simulink model "Guidance"  (R2021b)
settings: Solver=VariableStepAuto  StartTime=0.0  StopTime=10.0  RelTol=1e-3
settings Model: DataDictionary=GuidanceDD.sldd  Creator=camil  LastModifiedBy=Paul

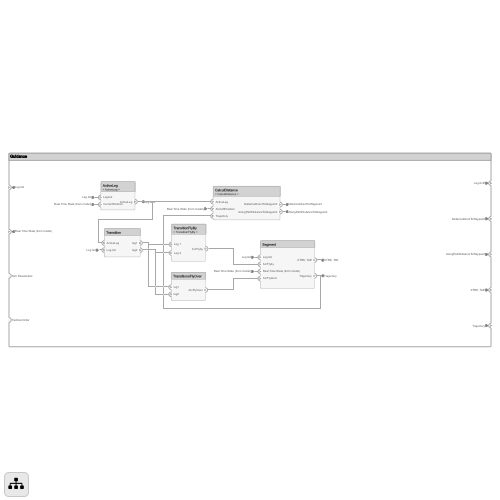
[thumbnail: Simulink's stored preview of the top-level diagram]
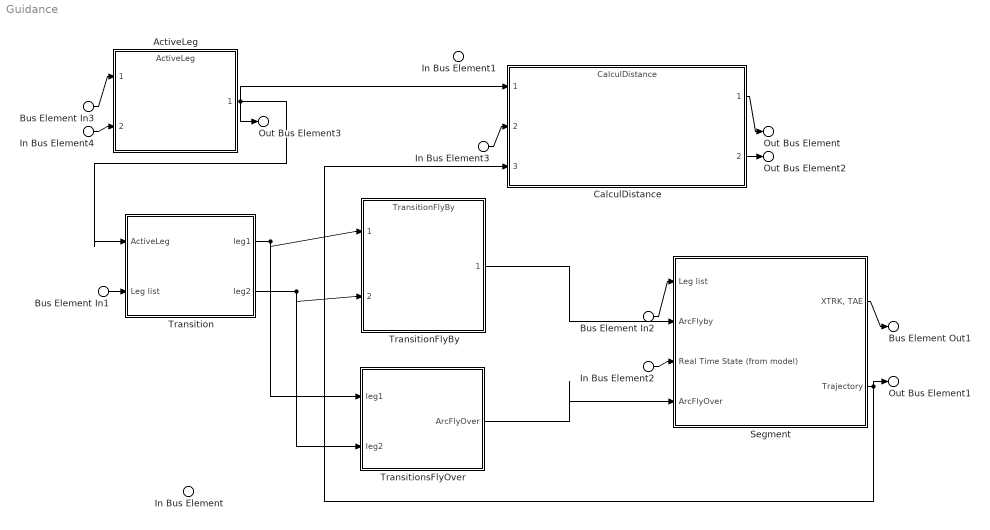
== system Guidance ==
  Bus Element In1 : Inport  RequirementInfo={} %GIDa_7ba553d4_af40_4941_a23b_14e6868a827f  PortName=Leg list
  Bus Element In2 : Inport  PortName=Leg list
  Bus Element In3 : Inport  PortName=Leg list
  In Bus Element3 : Inport  Port=2  PortName=Real Time State (from model)
  In Bus Element2 : Inport  Port=2  PortName=Real Time State (from model)
  In Bus Element4 : Inport  Port=2  PortName=Real Time State (from model)
  In Bus Element : Inport  Port=3  PortName=Sim Parameters
  In Bus Element1 : Inport  Port=4  PortName=Tactical Order
  ActiveLeg : ModelReference  ModelNameDialog=ActiveLeg.slx  SimulationMode=Normal  ModelReferenceVersion=1.2
      settings: PortSchema="{\"entries\":[{\"content\":{\"headerSize\":38,\"margin\":15,\"minimumSpacing\":25,\"sides\":[{\"content\":{\"connectorIds\":[\"In1\",\"In2\"]},\"type\":\"ConnectorPlacement.EquallySpacedRectSide\",\"uuid\":\"40658ef2-5221-47ab-ac15-ac3040122821\"},{\"content\":{\"connectorIds\":[\"Out1\"],\"side\":\"RIGHT\"},\"type\":\"ConnectorPlacement.EquallySpacedRectSide\",\"uuid\":\"9ff354e4-2199-4674-b496-2fe740e12343\"},{\"content\":{\"connectorIds\":[],\"side\":\"TOP\"},\"type\":\"ConnectorPlacement.EquallySpacedRectSide\",\"uuid\":\"dc5fc409-dad0-489a-b972-16c8f80e69f3\"}]},\"type\":\"ConnectorPlacement.EquallySpacedConnector\",\"uuid\":\"f90be94a-f4d5-4fcf-8904-697a887d48e1\"}],\"packageUris\":[\"http://schema.mathworks.com/mf0/Connector/R2020b\"],\"version\":\"1.0\"}"
  CalculDistance : ModelReference  ModelNameDialog=CalculDistance.slx  SimulationMode=Normal  ModelReferenceVersion=1.4
      settings: PortSchema="{\"entries\":[{\"content\":{\"headerSize\":38,\"margin\":15,\"minimumSpacing\":25,\"sides\":[{\"content\":{\"connectorIds\":[\"In1\",\"In2\",\"In3\"]},\"type\":\"ConnectorPlacement.EquallySpacedRectSide\",\"uuid\":\"40658ef2-5221-47ab-ac15-ac3040122821\"},{\"content\":{\"connectorIds\":[\"Out1\",\"Out2\"],\"side\":\"RIGHT\"},\"type\":\"ConnectorPlacement.EquallySpacedRectSide\",\"uuid\":\"9ff354e4-2199-4674-b496-2fe740e12343\"},{\"content\":{\"connectorIds\":[],\"side\":\"TOP\"},\"type\":\"ConnectorPlacement.EquallySpacedRectSide\",\"uuid\":\"dc5fc409-dad0-489a-b972-16c8f80e69f3\"}]},\"type\":\"ConnectorPlacement.EquallySpacedConnector\",\"uuid\":\"f90be94a-f4d5-4fcf-8904-697a887d48e1\"}],\"packageUris\":[\"http://schema.mathworks.com/mf0/Connector/R2020b\"],\"version\":\"1.0\"}"
  Segment : Subsystem
      settings: PortSchema="{\"entries\":[{\"content\":{\"headerSize\":26,\"margin\":15,\"minimumSpacing\":25,\"sides\":[{\"content\":{\"connectorIds\":[\"In1\",\"In2\",\"In3\",\"In4\"]},\"type\":\"ConnectorPlacement.EquallySpacedRectSide\",\"uuid\":\"6b59cfd3-505c-41dc-bf6c-4d82d451ef5d\"},{\"content\":{\"connectorIds\":[\"Out1\",\"Out2\"],\"side\":\"RIGHT\"},\"type\":\"ConnectorPlacement.EquallySpacedRectSide\",\"uuid\":\"f4142fc0-d8fd-40a0-bb01-f33d326facd2\"},{\"content\":{\"connectorIds\":[],\"side\":\"TOP\"},\"type\":\"ConnectorPlacement.EquallySpacedRectSide\",\"uuid\":\"178b855e-eaa2-4b70-a303-d3b7cb6a6ca3\"}]},\"type\":\"ConnectorPlacement.EquallySpacedConnector\",\"uuid\":\"50b576dd-2caa-4080-ba3f-9fa55a69b61e\"}],\"packageUris\":[\"http://schema.mathworks.com/mf0/Connector/R2020b\"],\"version\":\"1.0\"}"
  Transition : Subsystem
      settings: PortSchema="{\"entries\":[{\"content\":{\"headerSize\":26,\"margin\":15,\"minimumSpacing\":25,\"sides\":[{\"content\":{\"connectorIds\":[\"In1\",\"In2\"]},\"type\":\"ConnectorPlacement.EquallySpacedRectSide\",\"uuid\":\"1fe9f491-8940-4068-a798-04a3b940f4fc\"},{\"content\":{\"connectorIds\":[\"Out1\",\"Out2\"],\"side\":\"RIGHT\"},\"type\":\"ConnectorPlacement.EquallySpacedRectSide\",\"uuid\":\"599ca7dc-45bb-4841-abdf-2264bce8800e\"},{\"content\":{\"connectorIds\":[],\"side\":\"TOP\"},\"type\":\"ConnectorPlacement.EquallySpacedRectSide\",\"uuid\":\"c53441a1-491c-45f7-94f0-5f364038b604\"},{\"content\":{\"connectorIds\":[],\"side\":\"BOTTOM\"},\"type\":\"ConnectorPlacement.EquallySpacedRectSide\",\"uuid\":\"eccb86c1-1691-4b5e-892d-381328fb4de3\"}]},\"type\":\"ConnectorPlacement.EquallySpacedConnector\",\"uuid\":\"79cb965a-071d-4caa-a027-7b08a0e7657c\"}],\"packageUris\":[\"http://schema.mathworks.com/mf0/Connector/R2020b\"],\"version\":\"1.0\"}"
  TransitionFlyBy : ModelReference  ModelNameDialog=TransitionFlyBy.slx  SimulationMode=Normal  ModelReferenceVersion=1.5
      settings: PortSchema="{\"entries\":[{\"content\":{\"headerSize\":38,\"margin\":15,\"minimumSpacing\":25,\"sides\":[{\"content\":{\"connectorIds\":[\"In1\",\"In2\"]},\"type\":\"ConnectorPlacement.EquallySpacedRectSide\",\"uuid\":\"527312ce-8ecf-4bed-8b6c-5b5fdf65ac4f\"},{\"content\":{\"connectorIds\":[\"Out1\"],\"side\":\"RIGHT\"},\"type\":\"ConnectorPlacement.EquallySpacedRectSide\",\"uuid\":\"0e60a1e2-e39b-415d-9de3-d9c44bc8d6f1\"},{\"content\":{\"connectorIds\":[],\"side\":\"TOP\"},\"type\":\"ConnectorPlacement.EquallySpacedRectSide\",\"uuid\":\"eb1a168f-e7eb-4116-955a-7fd7ac806224\"}]},\"type\":\"ConnectorPlacement.EquallySpacedConnector\",\"uuid\":\"cb4b2f41-930a-4cb2-9ca3-9a6ca94f5e19\"}],\"packageUris\":[\"http://schema.mathworks.com/mf0/Connector/R2020b\"],\"version\":\"1.0\"}"
  TransitionsFlyOver : Subsystem
      settings: PortSchema="{\"entries\":[{\"content\":{\"headerSize\":26,\"margin\":15,\"minimumSpacing\":25,\"sides\":[{\"content\":{\"connectorIds\":[\"In1\",\"In2\"]},\"type\":\"ConnectorPlacement.EquallySpacedRectSide\",\"uuid\":\"1fe9f491-8940-4068-a798-04a3b940f4fc\"},{\"content\":{\"connectorIds\":[\"Out1\"],\"side\":\"RIGHT\"},\"type\":\"ConnectorPlacement.EquallySpacedRectSide\",\"uuid\":\"599ca7dc-45bb-4841-abdf-2264bce8800e\"},{\"content\":{\"connectorIds\":[],\"side\":\"TOP\"},\"type\":\"ConnectorPlacement.EquallySpacedRectSide\",\"uuid\":\"c53441a1-491c-45f7-94f0-5f364038b604\"}]},\"type\":\"ConnectorPlacement.EquallySpacedConnector\",\"uuid\":\"79cb965a-071d-4caa-a027-7b08a0e7657c\"}],\"packageUris\":[\"http://schema.mathworks.com/mf0/Connector/R2020b\"],\"version\":\"1.0\"}"
  Out Bus Element3 : Outport  PortName=Leg Actif
  Out Bus Element : Outport  Port=2  PortName=DistanceDirectToWaypoint
  Out Bus Element2 : Outport  Port=3  PortName=AlongPathDistanceToWaypoint
  Bus Element Out1 : Outport  RequirementInfo={} %GIDa_9dd73be6_6c5d_401c_be67_fba4302eb24d  Port=4  PortName=XTRK, TAE
  Out Bus Element1 : Outport  Port=5  PortName=Trajectory
  wires:
  Bus Element In1/1 -> Transition/2(Leg list)
  Transition/1(leg1) -> TransitionsFlyOver/1(leg1), TransitionFlyBy/1
  Transition/2(leg2) -> TransitionsFlyOver/2(leg2), TransitionFlyBy/2
  TransitionsFlyOver/1(ArcFlyOver) -> Segment/4(ArcFlyOver)
  Segment/2(Trajectory) -> Out Bus Element1/1, CalculDistance/3
  TransitionFlyBy/1 -> Segment/2(ArcFlyby)
  Bus Element In2/1 -> Segment/1(Leg list)
  In Bus Element2/1 -> Segment/3(Real Time State (from model))
  Segment/1("XTRK, TAE") -> Bus Element Out1/1
  In Bus Element3/1 -> CalculDistance/2
  CalculDistance/2 -> Out Bus Element2/1
  CalculDistance/1 -> Out Bus Element/1
  In Bus Element4/1 -> ActiveLeg/2
  Bus Element In3/1 -> ActiveLeg/1
  ActiveLeg/1 -> Transition/1(ActiveLeg), CalculDistance/1, Out Bus Element3/1

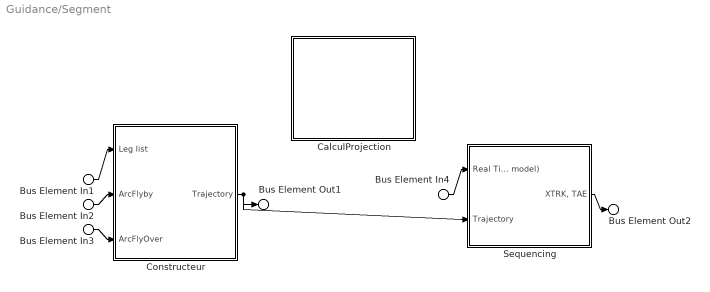
== system Guidance/Segment ==
  Bus Element In1 : Inport  PortName=Leg list
  Bus Element In2 : Inport  Port=2  PortName=ArcFlyby
  Bus Element In4 : Inport  Port=3  PortName=Real Time State (from model)
  Bus Element In3 : Inport  Port=4  PortName=ArcFlyOver
  CalculProjection : Subsystem
      settings: PortSchema="{\"entries\":[{\"content\":{\"headerSize\":26,\"margin\":15,\"minimumSpacing\":25,\"sides\":[{\"content\":{\"connectorIds\":[]},\"type\":\"ConnectorPlacement.EquallySpacedRectSide\",\"uuid\":\"6b59cfd3-505c-41dc-bf6c-4d82d451ef5d\"},{\"content\":{\"connectorIds\":[],\"side\":\"RIGHT\"},\"type\":\"ConnectorPlacement.EquallySpacedRectSide\",\"uuid\":\"f4142fc0-d8fd-40a0-bb01-f33d326facd2\"},{\"content\":{\"connectorIds\":[],\"side\":\"TOP\"},\"type\":\"ConnectorPlacement.EquallySpacedRectSide\",\"uuid\":\"178b855e-eaa2-4b70-a303-d3b7cb6a6ca3\"}]},\"type\":\"ConnectorPlacement.EquallySpacedConnector\",\"uuid\":\"50b576dd-2caa-4080-ba3f-9fa55a69b61e\"}],\"packageUris\":[\"http://schema.mathworks.com/mf0/Connector/R2020b\"],\"version\":\"1.0\"}"
  Constructeur : Subsystem
      settings: PortSchema="{\"entries\":[{\"content\":{\"headerSize\":26,\"margin\":15,\"minimumSpacing\":25,\"sides\":[{\"content\":{\"connectorIds\":[\"In1\",\"In2\",\"In3\"]},\"type\":\"ConnectorPlacement.EquallySpacedRectSide\",\"uuid\":\"1fe9f491-8940-4068-a798-04a3b940f4fc\"},{\"content\":{\"connectorIds\":[\"Out1\"],\"side\":\"RIGHT\"},\"type\":\"ConnectorPlacement.EquallySpacedRectSide\",\"uuid\":\"599ca7dc-45bb-4841-abdf-2264bce8800e\"},{\"content\":{\"connectorIds\":[],\"side\":\"TOP\"},\"type\":\"ConnectorPlacement.EquallySpacedRectSide\",\"uuid\":\"c53441a1-491c-45f7-94f0-5f364038b604\"}]},\"type\":\"ConnectorPlacement.EquallySpacedConnector\",\"uuid\":\"79cb965a-071d-4caa-a027-7b08a0e7657c\"}],\"packageUris\":[\"http://schema.mathworks.com/mf0/Connector/R2020b\"],\"version\":\"1.0\"}"
  Sequencing : Subsystem
      settings: PortSchema="{\"entries\":[{\"content\":{\"headerSize\":26,\"margin\":15,\"minimumSpacing\":25,\"sides\":[{\"content\":{\"connectorIds\":[\"In1\",\"In2\"]},\"type\":\"ConnectorPlacement.EquallySpacedRectSide\",\"uuid\":\"1fe9f491-8940-4068-a798-04a3b940f4fc\"},{\"content\":{\"connectorIds\":[\"Out1\"],\"side\":\"RIGHT\"},\"type\":\"ConnectorPlacement.EquallySpacedRectSide\",\"uuid\":\"599ca7dc-45bb-4841-abdf-2264bce8800e\"},{\"content\":{\"connectorIds\":[],\"side\":\"TOP\"},\"type\":\"ConnectorPlacement.EquallySpacedRectSide\",\"uuid\":\"c53441a1-491c-45f7-94f0-5f364038b604\"}]},\"type\":\"ConnectorPlacement.EquallySpacedConnector\",\"uuid\":\"79cb965a-071d-4caa-a027-7b08a0e7657c\"}],\"packageUris\":[\"http://schema.mathworks.com/mf0/Connector/R2020b\"],\"version\":\"1.0\"}"
  Bus Element Out2 : Outport  PortName=XTRK, TAE
  Bus Element Out1 : Outport  Port=2  PortName=Trajectory
  wires:
  Bus Element In1/1 -> Constructeur/1(Leg list)
  Bus Element In2/1 -> Constructeur/2(ArcFlyby)
  Bus Element In3/1 -> Constructeur/3(ArcFlyOver)
  Constructeur/1(Trajectory) -> Sequencing/2(Trajectory), Bus Element Out1/1
  Bus Element In4/1 -> Sequencing/1(Real Time State (from model))
  Sequencing/1("XTRK, TAE") -> Bus Element Out2/1

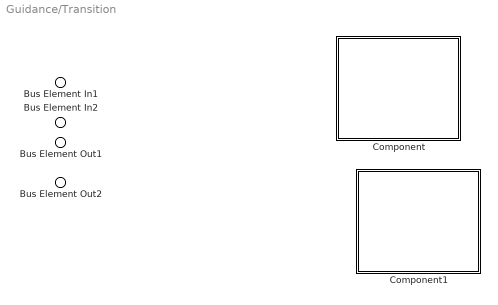
== system Guidance/Transition ==
  Bus Element In1 : Inport  PortName=ActiveLeg
  Bus Element In2 : Inport  Port=2  PortName=Leg list
  Component : Subsystem
      settings: PortSchema="{\"entries\":[{\"content\":{\"headerSize\":26,\"margin\":15,\"minimumSpacing\":25,\"sides\":[{\"content\":{\"connectorIds\":[]},\"type\":\"ConnectorPlacement.EquallySpacedRectSide\",\"uuid\":\"1fe9f491-8940-4068-a798-04a3b940f4fc\"},{\"content\":{\"connectorIds\":[],\"side\":\"RIGHT\"},\"type\":\"ConnectorPlacement.EquallySpacedRectSide\",\"uuid\":\"599ca7dc-45bb-4841-abdf-2264bce8800e\"},{\"content\":{\"connectorIds\":[],\"side\":\"TOP\"},\"type\":\"ConnectorPlacement.EquallySpacedRectSide\",\"uuid\":\"c53441a1-491c-45f7-94f0-5f364038b604\"}]},\"type\":\"ConnectorPlacement.EquallySpacedConnector\",\"uuid\":\"79cb965a-071d-4caa-a027-7b08a0e7657c\"}],\"packageUris\":[\"http://schema.mathworks.com/mf0/Connector/R2020b\"],\"version\":\"1.0\"}"
  Component1 : Subsystem
      settings: PortSchema="{\"entries\":[{\"content\":{\"headerSize\":26,\"margin\":15,\"minimumSpacing\":25,\"sides\":[{\"content\":{\"connectorIds\":[]},\"type\":\"ConnectorPlacement.EquallySpacedRectSide\",\"uuid\":\"1fe9f491-8940-4068-a798-04a3b940f4fc\"},{\"content\":{\"connectorIds\":[],\"side\":\"RIGHT\"},\"type\":\"ConnectorPlacement.EquallySpacedRectSide\",\"uuid\":\"599ca7dc-45bb-4841-abdf-2264bce8800e\"},{\"content\":{\"connectorIds\":[],\"side\":\"TOP\"},\"type\":\"ConnectorPlacement.EquallySpacedRectSide\",\"uuid\":\"c53441a1-491c-45f7-94f0-5f364038b604\"}]},\"type\":\"ConnectorPlacement.EquallySpacedConnector\",\"uuid\":\"79cb965a-071d-4caa-a027-7b08a0e7657c\"}],\"packageUris\":[\"http://schema.mathworks.com/mf0/Connector/R2020b\"],\"version\":\"1.0\"}"
  Bus Element Out1 : Outport  PortName=leg1
  Bus Element Out2 : Outport  Port=2  PortName=leg2

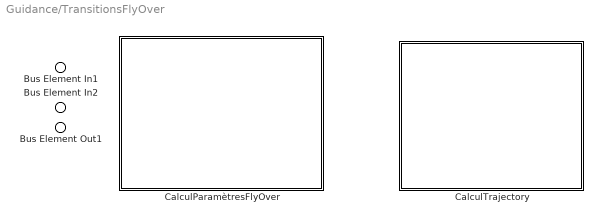
== system Guidance/TransitionsFlyOver ==
  Bus Element In1 : Inport  PortName=leg1
  Bus Element In2 : Inport  Port=2  PortName=leg2
  CalculParamètresFlyOver : Subsystem
      settings: PortSchema="{\"entries\":[{\"content\":{\"headerSize\":26,\"margin\":15,\"minimumSpacing\":25,\"sides\":[{\"content\":{\"connectorIds\":[]},\"type\":\"ConnectorPlacement.EquallySpacedRectSide\",\"uuid\":\"9778b81e-9a14-40e6-8857-e140a4abe5ee\"},{\"content\":{\"connectorIds\":[],\"side\":\"RIGHT\"},\"type\":\"ConnectorPlacement.EquallySpacedRectSide\",\"uuid\":\"d7e7a493-f06a-4f8b-8c78-1883ca79cab7\"},{\"content\":{\"connectorIds\":[],\"side\":\"TOP\"},\"type\":\"ConnectorPlacement.EquallySpacedRectSide\",\"uuid\":\"da95838c-2314-4569-b332-7fd5856dece2\"}]},\"type\":\"ConnectorPlacement.EquallySpacedConnector\",\"uuid\":\"a5fcad69-85d5-4a6e-b056-95e7f81e25a8\"}],\"packageUris\":[\"http://schema.mathworks.com/mf0/Connector/R2020b\"],\"version\":\"1.0\"}"
  CalculTrajectory : Subsystem
      settings: PortSchema="{\"entries\":[{\"content\":{\"headerSize\":26,\"margin\":15,\"minimumSpacing\":25,\"sides\":[{\"content\":{\"connectorIds\":[]},\"type\":\"ConnectorPlacement.EquallySpacedRectSide\",\"uuid\":\"6b59cfd3-505c-41dc-bf6c-4d82d451ef5d\"},{\"content\":{\"connectorIds\":[],\"side\":\"RIGHT\"},\"type\":\"ConnectorPlacement.EquallySpacedRectSide\",\"uuid\":\"f4142fc0-d8fd-40a0-bb01-f33d326facd2\"},{\"content\":{\"connectorIds\":[],\"side\":\"TOP\"},\"type\":\"ConnectorPlacement.EquallySpacedRectSide\",\"uuid\":\"178b855e-eaa2-4b70-a303-d3b7cb6a6ca3\"}]},\"type\":\"ConnectorPlacement.EquallySpacedConnector\",\"uuid\":\"50b576dd-2caa-4080-ba3f-9fa55a69b61e\"}],\"packageUris\":[\"http://schema.mathworks.com/mf0/Connector/R2020b\"],\"version\":\"1.0\"}"
  Bus Element Out1 : Outport  PortName=ArcFlyOver

== system Guidance/Segment/CalculProjection ==

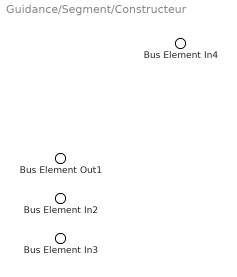
== system Guidance/Segment/Constructeur ==
  Bus Element In2 : Inport  PortName=Leg list
  Bus Element In4 : Inport  Port=2  PortName=ArcFlyby
  Bus Element In3 : Inport  Port=3  PortName=ArcFlyOver
  Bus Element Out1 : Outport  PortName=Trajectory

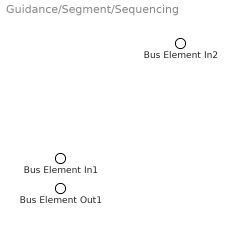
== system Guidance/Segment/Sequencing ==
  Bus Element In2 : Inport  PortName=Real Time State (from model)
  Bus Element In1 : Inport  Port=2  PortName=Trajectory
  Bus Element Out1 : Outport  PortName=XTRK, TAE

== system Guidance/Transition/Component ==

== system Guidance/Transition/Component1 ==

== system Guidance/TransitionsFlyOver/CalculParamètresFlyOver ==

== system Guidance/TransitionsFlyOver/CalculTrajectory ==
